simulink model "LinearPlanta1"  (Simulink 7.1)
settings: Solver=ode45  StartTime=0.0  StopTime=70  RelTol=1e-3
settings Model: Creator=ALUNO  LastModifiedBy=ALUNO
settings OptimizationCC: InlineInvariantSignals=on
settings DebuggingCC: SaveWithParameterizedLinksMsg=none  SignalResolutionControl=TryResolveAllWithWarning  MultiTaskDSMMsg=warning  MultiTaskCondExecSysMsg=none  StrictBusMsg=None
settings RTWCC: IncludeERTFirstTime=on
settings GRTTargetCC: TargetFcnLib=ansi_tfl_tmw.mat

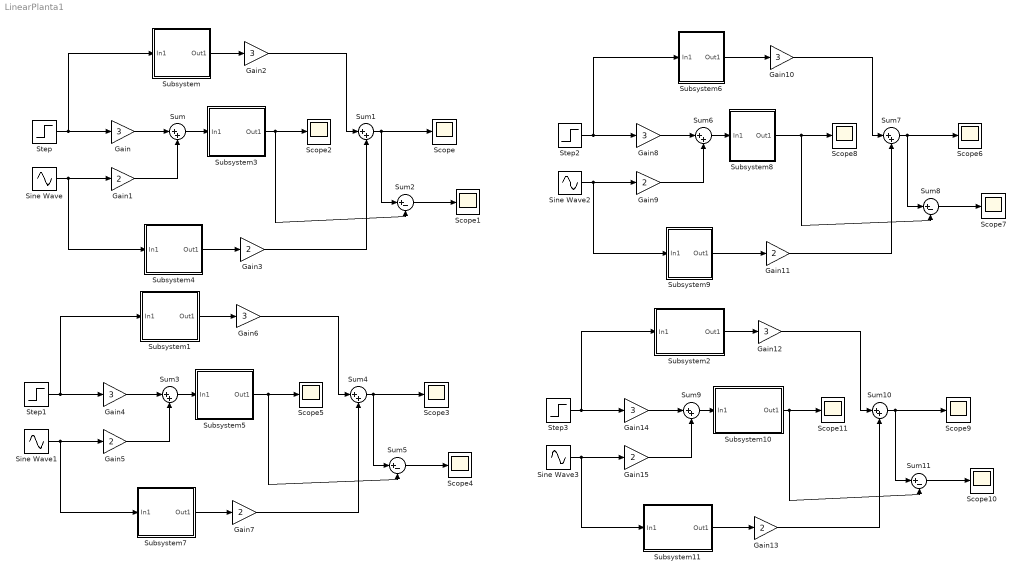
== system LinearPlanta1 ==
  Gain{,2,4,6,8,10,12,14} (8 alike) : Gain  Gain=3  ParameterDataType=sfix(16)  ParameterScaling=2^0  OutDataType=sfix(16)  OutScaling=2^0
  Gain{1,3,5,7,9,11,13,15} (8 alike) : Gain  Gain=2  ParameterDataType=sfix(16)  ParameterScaling=2^0  OutDataType=sfix(16)  OutScaling=2^0
  Scope{,1..11} (12 alike) : Scope
      Scope10 settings: SaveName=ScopeData9
      Scope11 settings: SaveName=ScopeData10
      Scope2 settings: SaveName=ScopeData2
      Scope3 settings: SaveName=ScopeData3
      Scope4 settings: SaveName=ScopeData4
      Scope5 settings: SaveName=ScopeData5
      Scope6 settings: SaveName=ScopeData6
      Scope7 settings: SaveName=ScopeData7
      Scope8 settings: SaveName=ScopeData8
      Scope9 settings: SaveName=ScopeData11
  Sine Wave{,1..3} (4 alike) : Sin  SampleTime=0
  Step{,1..3} (4 alike) : Step  SampleTime=0
  Subsystem : Subsystem
      mask Display: disp('Planta P1')
  Subsystem1 : Subsystem
      mask Display: disp('Planta P2')
  Subsystem10 : Subsystem
      mask Display: disp('Planta P4')
  Subsystem11 : Subsystem
      mask Display: disp('Planta P4')
  Subsystem2 : Subsystem
      mask Display: disp('Planta P4')
  Subsystem3 : Subsystem
      mask Display: disp('Planta P1')
  Subsystem4 : Subsystem
      mask Display: disp('Planta P1')
  Subsystem5 : Subsystem
      mask Display: disp('Planta P2')
  Subsystem6 : Subsystem
      mask Display: disp('Planta P3')
  Subsystem7 : Subsystem
      mask Display: disp('Planta P2')
  Subsystem8 : Subsystem
      mask Display: disp('Planta P3')
  Subsystem9 : Subsystem
      mask Display: disp('Planta P3')
  Sum{,1,3..4,6..7,9..10} (8 alike) : Sum  Inputs=|++  OutDataType=sfix(16)  OutScaling=2^0
  Sum{2,5,8,11} (4 alike) : Sum  Inputs=|+-  OutDataType=sfix(16)  OutScaling=2^0
  wires:
  Step/1 -> Gain/1, Subsystem/1(In1)
  Sine Wave/1 -> Gain1/1, Subsystem4/1(In1)
  Gain/1 -> Sum/1
  Gain1/1 -> Sum/2
  Sum/1 -> Subsystem3/1(In1)
  Subsystem3/1(Out1) -> Scope2/1, Sum2/2
  Subsystem/1(Out1) -> Gain2/1
  Subsystem4/1(Out1) -> Gain3/1
  Gain2/1 -> Sum1/1
  Gain3/1 -> Sum1/2
  Sum1/1 -> Scope/1, Sum2/1
  Sum2/1 -> Scope1/1
  Step1/1 -> Gain4/1, Subsystem1/1(In1)
  Sine Wave1/1 -> Gain5/1, Subsystem7/1(In1)
  Gain4/1 -> Sum3/1
  Gain5/1 -> Sum3/2
  Sum3/1 -> Subsystem5/1(In1)
  Subsystem5/1(Out1) -> Sum5/2, Scope5/1
  Subsystem1/1(Out1) -> Gain6/1
  Subsystem7/1(Out1) -> Gain7/1
  Gain6/1 -> Sum4/1
  Gain7/1 -> Sum4/2
  Sum4/1 -> Sum5/1, Scope3/1
  Sum5/1 -> Scope4/1
  Step2/1 -> Gain8/1, Subsystem6/1(In1)
  Sine Wave2/1 -> Gain9/1, Subsystem9/1(In1)
  Gain8/1 -> Sum6/1
  Gain9/1 -> Sum6/2
  Sum6/1 -> Subsystem8/1(In1)
  Subsystem8/1(Out1) -> Scope8/1, Sum8/2
  Subsystem6/1(Out1) -> Gain10/1
  Subsystem9/1(Out1) -> Gain11/1
  Gain10/1 -> Sum7/1
  Gain11/1 -> Sum7/2
  Sum7/1 -> Scope6/1, Sum8/1
  Sum8/1 -> Scope7/1
  Step3/1 -> Gain14/1, Subsystem2/1(In1)
  Sine Wave3/1 -> Gain15/1, Subsystem11/1(In1)
  Gain14/1 -> Sum9/1
  Gain15/1 -> Sum9/2
  Sum9/1 -> Subsystem10/1(In1)
  Subsystem10/1(Out1) -> Sum11/2, Scope11/1
  Subsystem2/1(Out1) -> Gain12/1
  Subsystem11/1(Out1) -> Gain13/1
  Gain12/1 -> Sum10/1
  Gain13/1 -> Sum10/2
  Sum10/1 -> Sum11/1, Scope9/1
  Sum11/1 -> Scope10/1

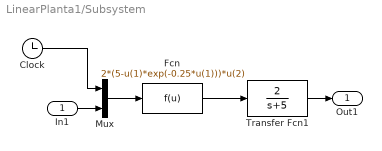
== system LinearPlanta1/Subsystem ==
  In1 : Inport  OutDataType=sfix(16)  OutScaling=2^0
  Clock : Clock
      settings: Decimation=10
  Fcn : Fcn  Expr=2*(5-u(1)*exp(-0.25*u(1)))*u(2)
  Mux : Mux  Inputs=2
  Transfer Fcn1 : TransferFcn  Numerator=[2]  Denominator=[1 5]
  Out1 : Outport  OutDataType=sfix(16)  OutScaling=2^0
  wires:
  Clock/1 -> Mux/1
  Mux/1 -> Fcn/1
  Fcn/1 -> Transfer Fcn1/1
  Transfer Fcn1/1 -> Out1/1
  In1/1 -> Mux/2

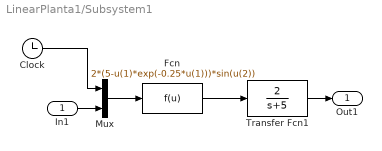
== system LinearPlanta1/Subsystem1 ==
  In1 : Inport  OutDataType=sfix(16)  OutScaling=2^0
  Clock : Clock
      settings: Decimation=10
  Fcn : Fcn  Expr=2*(5-u(1)*exp(-0.25*u(1)))*sin(u(2))
  Mux : Mux  Inputs=2
  Transfer Fcn1 : TransferFcn  Numerator=[2]  Denominator=[1 5]
  Out1 : Outport  OutDataType=sfix(16)  OutScaling=2^0
  wires:
  Clock/1 -> Mux/1
  Mux/1 -> Fcn/1
  Fcn/1 -> Transfer Fcn1/1
  Transfer Fcn1/1 -> Out1/1
  In1/1 -> Mux/2

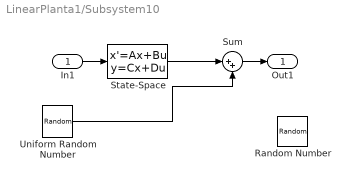
== system LinearPlanta1/Subsystem10 ==
  In1 : Inport  OutDataType=sfix(16)  OutScaling=2^0
  Random Number : RandomNumber  Variance=0.25  SampleTime=0
  State-Space : StateSpace  A=[-1 -2;1 0]  B=[1; 0]  C="[0  2]"  D=0
  Sum : Sum  Inputs=|++  OutDataType=sfix(16)  OutScaling=2^0
  Uniform Random Number : UniformRandomNumber  Minimum=-0.25  Maximum=0.25  SampleTime=0
  Out1 : Outport  OutDataType=sfix(16)  OutScaling=2^0
  wires:
  Uniform Random Number/1 -> Sum/2
  Sum/1 -> Out1/1
  In1/1 -> State-Space/1
  State-Space/1 -> Sum/1

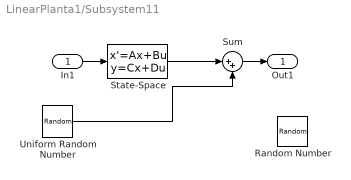
== system LinearPlanta1/Subsystem11 ==
  In1 : Inport  OutDataType=sfix(16)  OutScaling=2^0
  Random Number : RandomNumber  Variance=0.25  SampleTime=0
  State-Space : StateSpace  A=[-1 -2;1 0]  B=[1; 0]  C="[0  2]"  D=0
  Sum : Sum  Inputs=|++  OutDataType=sfix(16)  OutScaling=2^0
  Uniform Random Number : UniformRandomNumber  Minimum=-0.25  Maximum=0.25  SampleTime=0
  Out1 : Outport  OutDataType=sfix(16)  OutScaling=2^0
  wires:
  State-Space/1 -> Sum/1
  In1/1 -> State-Space/1
  Sum/1 -> Out1/1
  Uniform Random Number/1 -> Sum/2

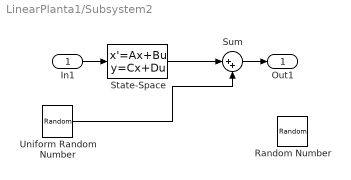
== system LinearPlanta1/Subsystem2 ==
  In1 : Inport  OutDataType=sfix(16)  OutScaling=2^0
  Random Number : RandomNumber  Variance=0.25  SampleTime=0
  State-Space : StateSpace  A=[-1 -2;1 0]  B=[1; 0]  C="[0  2]"  D=0
  Sum : Sum  Inputs=|++  OutDataType=sfix(16)  OutScaling=2^0
  Uniform Random Number : UniformRandomNumber  Minimum=-0.25  Maximum=0.25  SampleTime=0
  Out1 : Outport  OutDataType=sfix(16)  OutScaling=2^0
  wires:
  State-Space/1 -> Sum/1
  In1/1 -> State-Space/1
  Sum/1 -> Out1/1
  Uniform Random Number/1 -> Sum/2

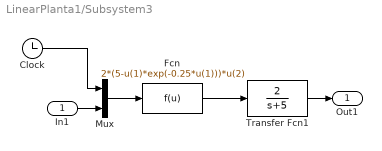
== system LinearPlanta1/Subsystem3 ==
  In1 : Inport  OutDataType=sfix(16)  OutScaling=2^0
  Clock : Clock
      settings: Decimation=10
  Fcn : Fcn  Expr=2*(5-u(1)*exp(-0.25*u(1)))*u(2)
  Mux : Mux  Inputs=2
  Transfer Fcn1 : TransferFcn  Numerator=[2]  Denominator=[1 5]
  Out1 : Outport  OutDataType=sfix(16)  OutScaling=2^0
  wires:
  Clock/1 -> Mux/1
  Mux/1 -> Fcn/1
  Fcn/1 -> Transfer Fcn1/1
  Transfer Fcn1/1 -> Out1/1
  In1/1 -> Mux/2

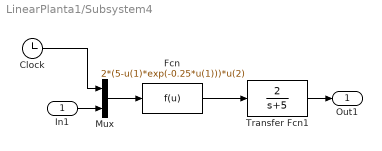
== system LinearPlanta1/Subsystem4 ==
  In1 : Inport  OutDataType=sfix(16)  OutScaling=2^0
  Clock : Clock
      settings: Decimation=10
  Fcn : Fcn  Expr=2*(5-u(1)*exp(-0.25*u(1)))*u(2)
  Mux : Mux  Inputs=2
  Transfer Fcn1 : TransferFcn  Numerator=[2]  Denominator=[1 5]
  Out1 : Outport  OutDataType=sfix(16)  OutScaling=2^0
  wires:
  Clock/1 -> Mux/1
  Mux/1 -> Fcn/1
  Fcn/1 -> Transfer Fcn1/1
  Transfer Fcn1/1 -> Out1/1
  In1/1 -> Mux/2

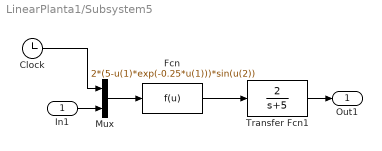
== system LinearPlanta1/Subsystem5 ==
  In1 : Inport  OutDataType=sfix(16)  OutScaling=2^0
  Clock : Clock
      settings: Decimation=10
  Fcn : Fcn  Expr=2*(5-u(1)*exp(-0.25*u(1)))*sin(u(2))
  Mux : Mux  Inputs=2
  Transfer Fcn1 : TransferFcn  Numerator=[2]  Denominator=[1 5]
  Out1 : Outport  OutDataType=sfix(16)  OutScaling=2^0
  wires:
  Clock/1 -> Mux/1
  Mux/1 -> Fcn/1
  Fcn/1 -> Transfer Fcn1/1
  Transfer Fcn1/1 -> Out1/1
  In1/1 -> Mux/2

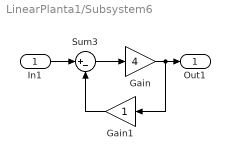
== system LinearPlanta1/Subsystem6 ==
  In1 : Inport  OutDataType=sfix(16)  OutScaling=2^0
  Gain : Gain  Gain=4  ParameterDataType=sfix(16)  ParameterScaling=2^0  OutDataType=sfix(16)  OutScaling=2^0
  Gain1 : Gain  Orientation=left  ParameterDataType=sfix(16)  ParameterScaling=2^0  OutDataType=sfix(16)  OutScaling=2^0
  Sum3 : Sum  Inputs=|+-  OutDataType=sfix(16)  OutScaling=2^0
  Out1 : Outport  OutDataType=sfix(16)  OutScaling=2^0
  wires:
  Sum3/1 -> Gain/1
  Gain1/1 -> Sum3/2
  Gain/1 -> Out1/1, Gain1/1
  In1/1 -> Sum3/1

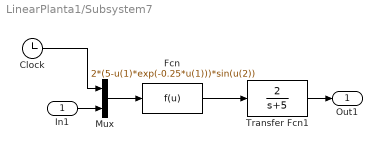
== system LinearPlanta1/Subsystem7 ==
  In1 : Inport  OutDataType=sfix(16)  OutScaling=2^0
  Clock : Clock
      settings: Decimation=10
  Fcn : Fcn  Expr=2*(5-u(1)*exp(-0.25*u(1)))*sin(u(2))
  Mux : Mux  Inputs=2
  Transfer Fcn1 : TransferFcn  Numerator=[2]  Denominator=[1 5]
  Out1 : Outport  OutDataType=sfix(16)  OutScaling=2^0
  wires:
  In1/1 -> Mux/2
  Transfer Fcn1/1 -> Out1/1
  Fcn/1 -> Transfer Fcn1/1
  Mux/1 -> Fcn/1
  Clock/1 -> Mux/1

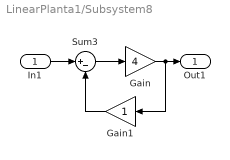
== system LinearPlanta1/Subsystem8 ==
  In1 : Inport  OutDataType=sfix(16)  OutScaling=2^0
  Gain : Gain  Gain=4  ParameterDataType=sfix(16)  ParameterScaling=2^0  OutDataType=sfix(16)  OutScaling=2^0
  Gain1 : Gain  Orientation=left  ParameterDataType=sfix(16)  ParameterScaling=2^0  OutDataType=sfix(16)  OutScaling=2^0
  Sum3 : Sum  Inputs=|+-  OutDataType=sfix(16)  OutScaling=2^0
  Out1 : Outport  OutDataType=sfix(16)  OutScaling=2^0
  wires:
  In1/1 -> Sum3/1
  Gain/1 -> Gain1/1, Out1/1
  Gain1/1 -> Sum3/2
  Sum3/1 -> Gain/1

== system LinearPlanta1/Subsystem9 ==
  In1 : Inport  OutDataType=sfix(16)  OutScaling=2^0
  Gain : Gain  Gain=4  ParameterDataType=sfix(16)  ParameterScaling=2^0  OutDataType=sfix(16)  OutScaling=2^0
  Gain1 : Gain  Orientation=left  ParameterDataType=sfix(16)  ParameterScaling=2^0  OutDataType=sfix(16)  OutScaling=2^0
  Sum3 : Sum  Inputs=|+-  OutDataType=sfix(16)  OutScaling=2^0
  Out1 : Outport  OutDataType=sfix(16)  OutScaling=2^0
  wires:
  Sum3/1 -> Gain/1
  Gain1/1 -> Sum3/2
  Gain/1 -> Out1/1, Gain1/1
  In1/1 -> Sum3/1
